simulink model "q6_H_inf_sim"  (R2019a)
settings: Solver=VariableStepAuto  StartTime=0.0  StopTime=T  RelTol=1e-3
values from neighbouring files (symbols this model uses):
  A = [0 0 0 1 0 0 ... (first row only)    [q5_LQR_and_H_infinty.m]
  B1h = [0 0 0 0 1/m2 0]'    [q5_LQR_and_H_infinty.m]
  B2h = [0 0 0 1/m1 0 0]'    [q5_LQR_and_H_infinty.m]
  C = [0 0 1 0 0 0]    [q5_LQR_and_H_infinty.m]
  Kh = inv(gama1_h)*B2h'*Ph    [q5_LQR_and_H_infinty.m]
settings Model: Creator=ronil  LastModifiedBy=ronil

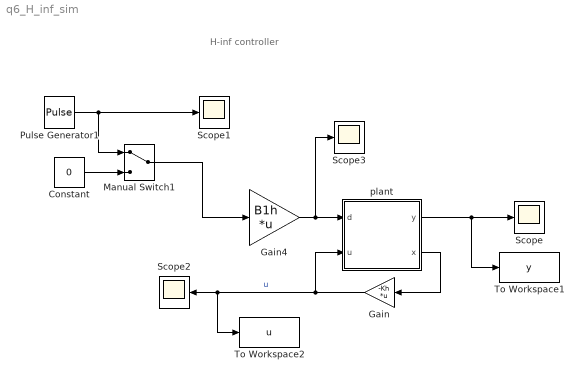
== system q6_H_inf_sim ==
  note: H-inf controller
  Constant : Constant  Value=0
  Gain : Gain  Gain=-Kh  Multiplication=Matrix(K*u)
  Gain4 : Gain  Gain=B1h  Multiplication=Matrix(K*u)
  Manual Switch1 : ManualSwitch
  Pulse Generator1 : DiscretePulseGenerator  PulseType=Time based  Amplitude=10  Period=10  PulseWidth=5
  Scope{,1..3} (4 alike) : Scope
  To Workspace1 : ToWorkspace  VariableName=y  SaveFormat=Timeseries  SampleTime=-1
  To Workspace2 : ToWorkspace  VariableName=u  SaveFormat=Timeseries  SampleTime=-1
  plant : Subsystem
  wires:
  Gain/1 -> plant/2(u), Scope2/1, To Workspace2/1  "u"
  Manual Switch1/1 -> Gain4/1
  plant/1(y) -> To Workspace1/1, Scope/1
  Gain4/1 -> Scope3/1, plant/1(d)
  plant/2(x) -> Gain/1
  Constant/1 -> Manual Switch1/2
  Pulse Generator1/1 -> Scope1/1, Manual Switch1/1

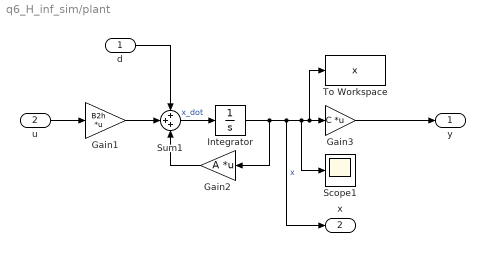
== system q6_H_inf_sim/plant ==
  d : Inport
  u : Inport  Port=2
  Gain1 : Gain  Gain=B2h  Multiplication=Matrix(K*u)
  Gain2 : Gain  Gain=A  Multiplication=Matrix(K*u)
  Gain3 : Gain  Gain=C  Multiplication=Matrix(K*u)
  Integrator : Integrator  InitialCondition=[0 0 0 0 0 0]
  Scope1 : Scope
  Sum1 : Sum  Inputs=+++
  To Workspace : ToWorkspace  VariableName=x  SaveFormat=Timeseries  SampleTime=-1
  y : Outport
  x : Outport  Port=2
  wires:
  d/1 -> Sum1/1
  Gain1/1 -> Sum1/2
  Gain2/1 -> Sum1/3
  Integrator/1 -> x/1, Scope1/1, To Workspace/1, Gain3/1, Gain2/1  "x"
  Sum1/1 -> Integrator/1  "x_dot"
  Gain3/1 -> y/1
  u/1 -> Gain1/1
